simulink model "testMaster"  (R2022a)
settings: Solver=VariableStepAuto  StartTime=0.0  StopTime=10  RelTol=1e-3
values from neighbouring files (symbols this model uses):
  dt = ds/v    [DefineUAVPath.m]    (also in DronePathPlanSubsystem.m; PathPlanSubsystem.m = ds/speed)
undefined symbols (not defined in the file or in its folder): Env
libraries: aerolibanimutils x2
settings Model: Creator=zckog  LastModifiedBy=zckog
settings DebuggingCC: UnconnectedInputMsg=warning  UnconnectedOutputMsg=warning  UnconnectedLineMsg=warning
settings RTWCC: DLArmComputeVersion=19.05

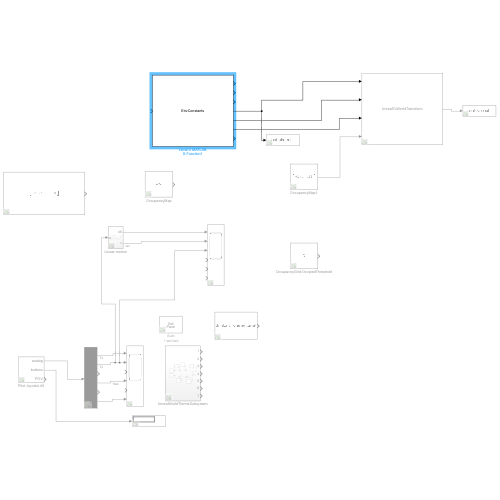
[thumbnail: Simulink's stored preview of the top-level diagram]
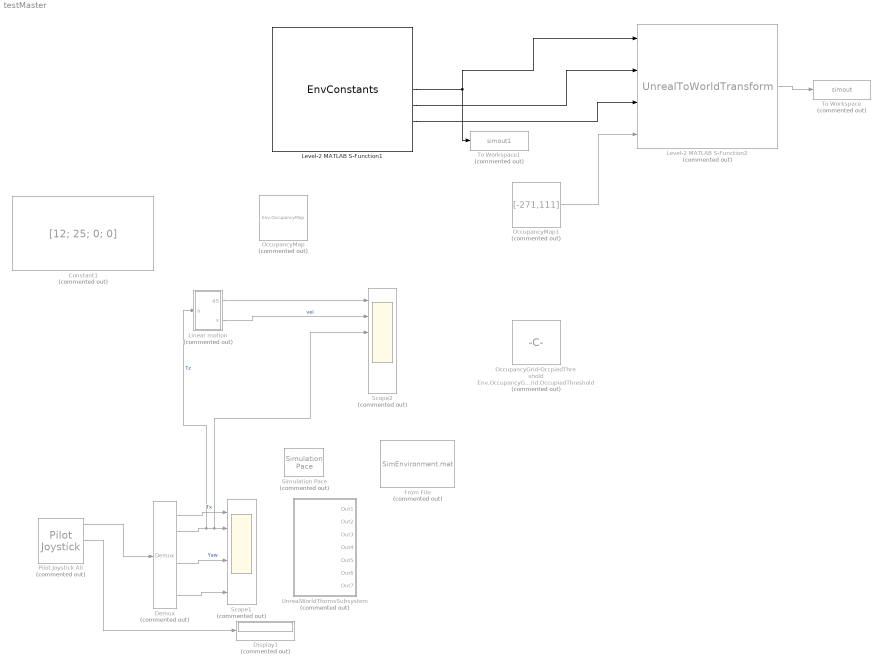
== system testMaster ==
  Constant1 : Constant  Commented=on  Value=[12; 25; 0; 0]  OutDataTypeStr=int32  SampleTime=1
  Demux : Demux  Commented=on  Outputs=6
  Display1 : Display  Commented=on
  From File : FromFile  Commented=on  FileName=SimEnvironment.mat  SampleTime=0
  Level-2 MATLAB S-Function1 : M-S-Function  Priority=1  FunctionName=EnvConstants
  Level-2 MATLAB S-Function2 : M-S-Function  Priority=1  Commented=on  FunctionName=UnrealToWorldTransform
  Linear motion : Subsystem  Commented=on
  OccupancyGrid-OccpiedThreshold : Constant  Commented=on  Value=Env.OccupancyGrid.OccupiedThreshold
  OccupancyMap : Constant  Commented=on  Value=Env.OccupancyMap
  OccupancyMap1 : Constant  Commented=on  Value=[-271,111]  OutDataTypeStr=single
  Pilot Joystick All : aerolibanimutils/Pilot Joystick  Commented=on  JoystickID=Joystick1  OutputConfiguration=AllOutputs  SampleTime=dt
  Scope1 : Scope  Commented=on  NumInputPorts=6
  Scope2 : Scope  Commented=on  NumInputPorts=6
  Simulation Pace : aerolibanimutils/Simulation Pace  Commented=on  SimulationPace=1  SleepMode=Auto  OutputPaceError=off  SampleTime=dt
  To Workspace : ToWorkspace  Commented=on  VariableName=simout  SaveFormat=Timeseries  SampleTime=-1
  To Workspace1 : ToWorkspace  Commented=on  VariableName=simout1  SaveFormat=Timeseries  SampleTime=-1
  UnrealWorldTformsSubsystem : Subsystem  Commented=on
  wires:
  Pilot Joystick All/1 -> Demux/1
  Demux/2 -> Linear motion/1(a), Scope2/3, Scope1/2  "Tz"
  Demux/1 -> Scope1/1  "Tx"
  Demux/4 -> Scope1/4  "Yaw"
  Demux/6 -> Scope1/6
  Pilot Joystick All/2 -> Display1/1
  Linear motion/1(dS) -> Scope2/1
  Linear motion/2(v) -> Scope2/2  "vel"
  OccupancyMap1/1 -> Level-2 MATLAB S-Function2/4
  Level-2 MATLAB S-Function1/4 -> Level-2 MATLAB S-Function2/1, To Workspace1/1
  Level-2 MATLAB S-Function1/5 -> Level-2 MATLAB S-Function2/2
  Level-2 MATLAB S-Function1/6 -> Level-2 MATLAB S-Function2/3
  Level-2 MATLAB S-Function2/1 -> To Workspace/1

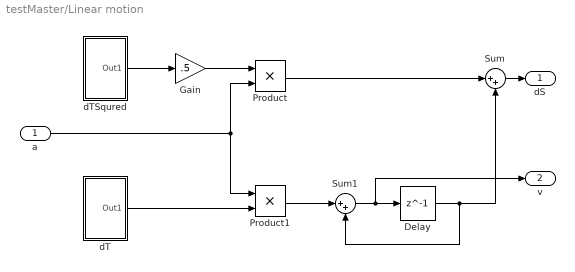
== system testMaster/Linear motion ==
  a : Inport
  Delay : Delay  DelayLength=1  InitialCondition=0
  Gain : Gain  Gain=.5
  Product : Product
  Product1 : Product
  Sum : Sum  Inputs=|++
  Sum1 : Sum  Inputs=|++
  dT : Subsystem
  dTSqured : Subsystem
  dS : Outport
  v : Outport  Port=2
  wires:
  a/1 -> Product/2, Product1/1
  Product1/1 -> Sum1/1
  Delay/1 -> Sum/2, Sum1/2
  dTSqured/1(Out1) -> Gain/1
  Product/1 -> Sum/1
  Gain/1 -> Product/1
  dT/1(Out1) -> Product1/2
  Sum/1 -> dS/1
  Sum1/1 -> v/1, Delay/1

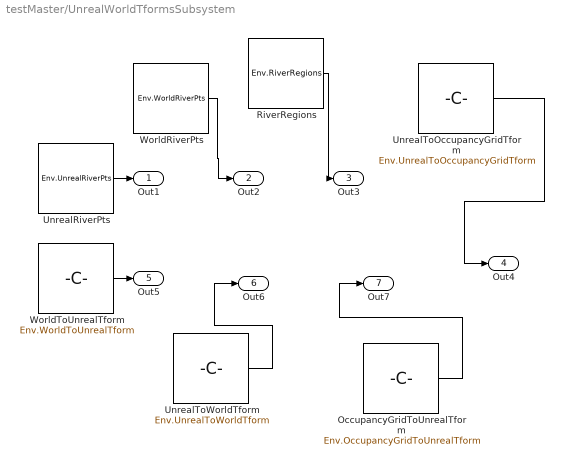
== system testMaster/UnrealWorldTformsSubsystem ==
  OccupancyGridToUnrealTform : Constant  Value=Env.OccupancyGridToUnrealTform
  RiverRegions : Constant  Value=Env.RiverRegions
  UnrealRiverPts : Constant  Value=Env.UnrealRiverPts
  UnrealToOccupancyGridTform : Constant  Value=Env.UnrealToOccupancyGridTform
  UnrealToWorldTform : Constant  Value=Env.UnrealToWorldTform
  WorldRiverPts : Constant  Value=Env.WorldRiverPts
  WorldToUnrealTform : Constant  Value=Env.WorldToUnrealTform
  Out1 : Outport
  Out2 : Outport  Port=2
  Out3 : Outport  Port=3
  Out4 : Outport  Port=4
  Out5 : Outport  Port=5
  Out6 : Outport  Port=6
  Out7 : Outport  Port=7
  wires:
  UnrealToOccupancyGridTform/1 -> Out4/1
  UnrealToWorldTform/1 -> Out6/1
  UnrealRiverPts/1 -> Out1/1
  WorldRiverPts/1 -> Out2/1
  OccupancyGridToUnrealTform/1 -> Out7/1
  WorldToUnrealTform/1 -> Out5/1
  RiverRegions/1 -> Out3/1

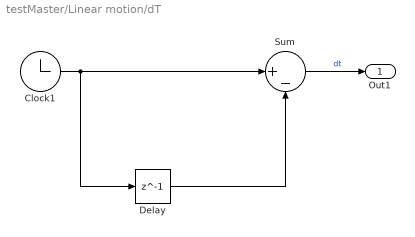
== system testMaster/Linear motion/dT ==
  Clock1 : Clock
  Delay : Delay  DelayLength=1  InitialCondition=0
  Sum : Sum  Inputs=|+-
  Out1 : Outport
  wires:
  Sum/1 -> Out1/1  "dt"
  Clock1/1 -> Sum/1, Delay/1
  Delay/1 -> Sum/2

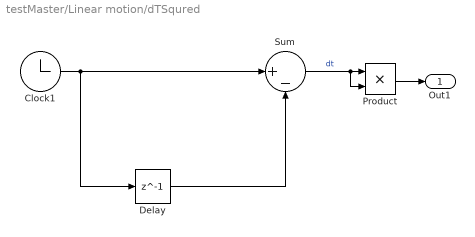
== system testMaster/Linear motion/dTSqured ==
  Clock1 : Clock
  Delay : Delay  DelayLength=1  InitialCondition=0
  Product : Product
  Sum : Sum  Inputs=|+-
  Out1 : Outport
  wires:
  Sum/1 -> Product/2, Product/1  "dt"
  Clock1/1 -> Sum/1, Delay/1
  Delay/1 -> Sum/2
  Product/1 -> Out1/1
